simulink model "Task_1"  (R2016a)
settings: Solver=VariableStepAuto  StartTime=0.0  StopTime=5  RelTol=1e-3
libraries: dspsrcs4 x2
settings Model: Creator=92301  LastModifiedBy=92301

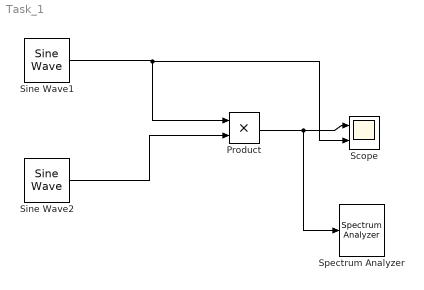
== system Task_1 ==
  Product : Product
  Scope : Scope  NumInputPorts=2
  "Sine Wave1 " : dspsrcs4/Sine Wave  Amplitude=5  Frequency=10  Phase=0  SampleMode=Discrete  OutComplex=Real  CompMethod=Trigonometric fcn  TableSize=Speed  SampleTime=1/1000  SamplesPerFrame=1  ResetState=Restart at time zero  OutputFrames=off  dataType=double  wordLen=16  udDataType=sfix(16)  fracBitsMode=Best precision  numFracBits=15  OutDataTypeStr=double  LastOutDataTypeStr=double
  "Sine Wave2 " : dspsrcs4/Sine Wave  Amplitude=5  Frequency=100  Phase=0  SampleMode=Discrete  OutComplex=Real  CompMethod=Trigonometric fcn  TableSize=Speed  SampleTime=1/1000  SamplesPerFrame=1  ResetState=Restart at time zero  OutputFrames=off  dataType=double  wordLen=16  udDataType=sfix(16)  fracBitsMode=Best precision  numFracBits=15  OutDataTypeStr=double  LastOutDataTypeStr=double
  Spectrum Analyzer : SpectrumAnalyzer
  wires:
  "Sine Wave1 "/1 -> Scope/2, Product/1
  "Sine Wave2 "/1 -> Product/2
  Product/1 -> Spectrum Analyzer/1, Scope/1
